simulink model "Final_Simulation_unfiltered_speed"  (R2024b)
settings: Solver=VariableStepAuto  StartTime=0.0  StopTime=30  MaxStep=1e-4  RelTol=1e-4
libraries: spsDiodeLib x7, spsVoltageMeasurementLib x5, spsCurrentMeasurementLib x4, spsControlledVoltageSourceLib x3, spsDCMachineLib x1, spsDCVoltageSourceLib x1, spsGroundLib x1, spsMosfetLib x1, slpidlib x1, spsPWMGeneratorDCDCLib x1, spsRMSLib x1, spsSeriesRLCBranchLib x1
settings Model: Creator=sefer  LastModifiedBy=PC
settings DebuggingCC: IgnoredZcDiagnostic=none

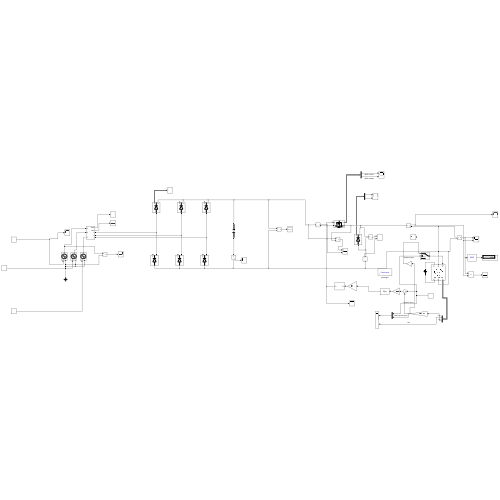
[thumbnail: Simulink's stored preview of the top-level diagram]
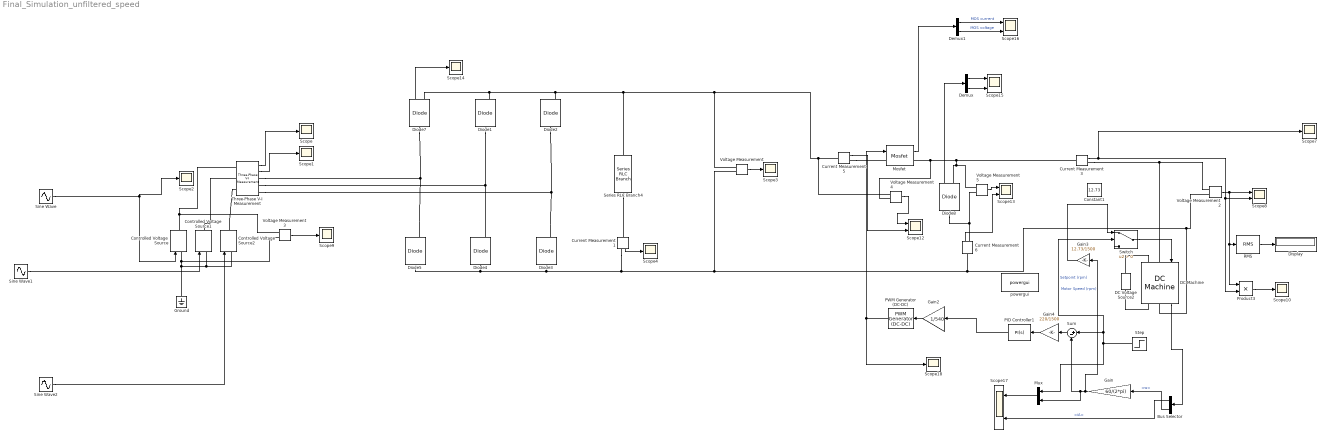
== system Final_Simulation_unfiltered_speed ==
  Bus Selector : BusSelector  OutputSignals=iA,w
  Constant1 : Constant  Value=12.73
  Controlled Voltage Source : spsControlledVoltageSourceLib/Controlled Voltage Source  Initialize=on  Source_Type=AC  Amplitude=0  Phase=0  Frequency=50  Measurements=None
  Controlled Voltage Source1 : spsControlledVoltageSourceLib/Controlled Voltage Source  Initialize=on  Source_Type=AC  Amplitude=0  Phase=0  Frequency=50  Measurements=None
  Controlled Voltage Source2 : spsControlledVoltageSourceLib/Controlled Voltage Source  Initialize=on  Source_Type=AC  Amplitude=0  Phase=0  Frequency=50  Measurements=None
  Current Measurement{1,3,5..6} (4 alike) : spsCurrentMeasurementLib/Current Measurement  PhasorSimulation=off  OutputType=Complex  PSBequivalent=0
  DC Machine : spsDCMachineLib/DC Machine  PresetModel=No  MechanicalLoad=Torque TL  FieldType=Wound  ShowDetailedParameters=on  MeasurementBus=on  RLa="[ 0.8  12.5e-3]"  RLf="[210  23]"  Laf=1.3  MachineConstant=Torque constant (N.m/A)  Ke=1.8  Kt=1.8  J=0.2  Bm=0.005  Tf=0  w0=0  Ifinit=1.04761904761905  TsPowergui=0  TsBlock=-1
  DC Voltage Source2 : spsDCVoltageSourceLib/DC Voltage Source  Amplitude=220  Measurements=None
  Demux : Demux  Outputs=2
  Demux1 : Demux  Outputs=2
  Diode{1..5,7} (6 alike) : spsDiodeLib/Diode  Ron=0.001  Lon=0  Vf=0  IC=0  UseSnubber=0  Rs=inf  Cs=0  Measurements=on
  Diode8 : spsDiodeLib/Diode  Ron=0  Lon=0  Vf=0  IC=0  UseSnubber=0  Rs=inf  Cs=0  Measurements=on
  Display : Display
  Gain : Gain  Gain=60/(2*pi)
  Gain2 : Gain  Gain=1/540
  Gain3 : Gain  Gain=12.73/1500
  Gain4 : Gain  Gain=220/1500
  Ground : spsGroundLib/Ground  LConnTagsString=a
  Mosfet : spsMosfetLib/Mosfet  Ron=0.1  Lon=0  Rd=0.01  Vfd=0  IC=0  Rs=1e5  Cs=inf  Measurements=on
  Mux : Mux  Inputs=2
  PID Controller1 : slpidlib/PID Controller  Controller=PI  Form=Parallel  TimeDomain=Continuous-time  UseExternalTs=off  SampleTime=-1  IntegratorMethod=Forward Euler  FilterMethod=Forward Euler  ControllerParametersSource=internal  P=0.01  I=0.28994889807594  UseKiTs=off  D=-0.000982857561820016  UseExternalDerivativeSource=off  N=2.14059506099866  UseFilter=on  TunerSelectOption=Transfer Function Based (PID Tuner App)  InitialConditionSource=internal  InitialConditionForIntegrator=0  InitialConditionForFilter=0  DifferentiatorICPrevScaledInput=0  ExternalReset=none  TrackingMode=off  Kt=1  LimitOutput=off  SatLimitsSource=internal  UpperSaturationLimit=100  LowerSaturationLimit=-100  LinearizeAsGain=on  AntiWindupMode=none  Kb=1  LimitIntegrator=on  UpperIntegratorSaturationLimit=1500  LowerIntegratorSaturationLimit=-1500  POutMin=[]  POutMax=[]  IOutMin=[]  IOutMax=[]  DOutMin=[]  DOutMax=[]  NOutMin=[]  NOutMax=[]  SumOutMin=[]  SumOutMax=[]  SaturationOutMin=[]  SaturationOutMax=[]  PParamMin=[]  PParamMax=[]  IParamMin=[]  IParamMax=[]  DParamMin=[]  DParamMax=[]  NParamMin=[]  NParamMax=[]  KbParamMin=[]  KbParamMax=[]  KtParamMin=[]  KtParamMax=[]  KbOutMin=[]  KbOutMax=[]  KtOutMin=[]  KtOutMax=[]  IntegratorOutMin=[]  IntegratorOutMax=[]  FilterOutMin=[]  FilterOutMax=[]  SumI1OutMin=[]  SumI1OutMax=[]  SumI2OutMin=[]  SumI2OutMax=[]  SumI3OutMin=[]  SumI3OutMax=[]  SumI4OutMin=[]  SumI4OutMax=[]  SumDOutMin=[]  SumDOutMax=[]  DifferentiatorOutMin=[]  DifferentiatorOutMax=[]  FilterDiffOutCoefMin=[]  FilterDiffOutCoefMax=[]  ReciprocalOutMin=[]  ReciprocalOutMax=[]  SumDenOutMin=[]  SumDenOutMax=[]  SumNumOutMin=[]  SumNumOutMax=[]  DivideOutMin=[]  DivideOutMax=[]  UdiffTsProdOutMin=[]  UdiffTsProdOutMax=[]  NTsProdOutMin=[]  NTsProdOutMax=[]  UintegralTsProdOutMin=[]  UintegralTsProdOutMax=[]  UngainTsProdOutMin=[]  UngainTsProdOutMax=[]  ClampingZeroOutDataTypeStr=Inherit: Inherit via back propagation  ClampingZeroOutMin=[]  ClampingZeroOutMax=[]  FilterDenConstantOutDataTypeStr=Inherit: Inherit via back propagation  FilterDenConstantOutMin=[]  FilterDenConstantOutMax=[]  PCopyOutDataTypeStr=Inherit: Inherit via back propagation  PCopyOutMin=[]  PCopyOutMax=[]  NCopyOutDataTypeStr=Inherit: Inherit via back propagation  NCopyOutMin=[]  NCopyOutMax=[]  IntegratorContinuousStateAttributes=''  IntegratorStateMustResolveToSignalObject=off  IntegratorRTWStateStorageClass=Auto  FilterContinuousStateAttributes=''  FilterStateMustResolveToSignalObject=off  FilterRTWStateStorageClass=Auto  ParallelPVariant=InternalParameters  IdealPVariant=Disabled  IVariant=InternalParameters  DVariant=Disabled  IntegratorVariant=Continuous  SatVariant=Disabled  AWVariant=Passthrough  PCopyVariant=Disabled  TRVariant=Disabled  FdbkBlocksVariant=Forward  IdealPFdbkVariant=Disabled  SatFdbkVariant=Disabled  DerivativeFilterVariant=Disabled  NVariant=Disabled  NCopyVariant=Disabled_SignalSpec  FilterICVariant=Disabled  IntegratorICVariant=InternalICs  ExternalResetVariant=Disabled  TRSumVariant=Passthrough  SumFdbkVariant=Disabled  SumVariant=Sum_PI  TsampFilterVariant=InternalTs  TsampNgainVariant=Passthrough  TsampIntegralVariant=Disabled_SignalSpec  ExternalSaturationOutDataTypeStr=Inherit: Same as second input  DerivativeSourceVariant=Disabled  PreIntVariant=InternalPreInt
  PWM Generator (DC-DC) : spsPWMGeneratorDCDCLib/PWM Generator (DC-DC)  Fsw=5000  Ts=0
  Product3 : Product
  RMS : spsRMSLib/RMS  TrueRMS=on  Freq=60  RMSInit=120  Ts=0
  Scope{,1..4,7,9..10,14,18} (10 alike) : Scope
  Scope{8,12..13,15..17} (6 alike) : Scope  NumInputPorts=2
  Series RLC Branch4 : spsSeriesRLCBranchLib/Series RLC Branch  LConnTagsString=__new0  RConnTagsString=__new0  BranchType=C  Resistance=0.001  Inductance=1e-3  SetiL0=off  InitialCurrent=0  Capacitance=2000e-6  Setx0=off  InitialVoltage=0  Measurements=None
  Sine Wave : Sin  Amplitude=230*sqrt(2)  Frequency=100*pi  SampleTime=0
  Sine Wave1 : Sin  Amplitude=230*sqrt(2)  Frequency=100*pi  Phase=2*pi/3  SampleTime=0
  Sine Wave2 : Sin  Amplitude=230*sqrt(2)  Frequency=100*pi  Phase=4*pi/3  SampleTime=0
  Step : Step  After=1500  SampleTime=0
  Sum : Sum  Inputs=|+-
  Switch : Switch  Criteria=u2 > Threshold  SaturateOnIntegerOverflow=off  InputSameDT=off
  Three-Phase V-I Measurement : spsThreePhaseVIMeasurementLib/Three-Phase V-I Measurement  VoltageMeasurement=phase-to-ground  SetLabelV=off  LabelV=Vabc  Vpu=off  VpuLL=off  CurrentMeasurement=yes  SetLabelI=off  LabelI=Iabc  Ipu=off  Pbase=100e6  Vbase=500e3  OutputType=Complex  PhasorSimulation=off  PSBequivalent=0
  Voltage Measurement{,2..5} (5 alike) : spsVoltageMeasurementLib/Voltage Measurement  PhasorSimulation=off  OutputType=Complex  PSBequivalent=0
  powergui : sps_lib/powergui  Priority=1  SimulationMode=Continuous  SampleTime=1e-6  frequency=60  Iterations=50  frequencyindice=0  Pbase=100e6  ErrMax=1e-4  UnitsV=kV  UnitsW=MW  buscounter=0  FunctionMessages=off  echomessages=off  EnableUseOfTLC=off  CurrentSourceSwitches=off  DisableSnubberDevices=off  DisableRonSwitches=off  DisableVfSwitches=off  DisplayEquations=off  AutomaticDiscreteSolvers=off  SolverType=Tustin/Backward Euler (TBE)  Interpol=off  ExternalGateDelay=off  methode=off  Ts=100  x0status=blocks  SPID=on  SwTol=0  HookPort=off  NonlinearTolerance=1e-4  nMaxIteration=100  ContinueOnMaxIteration=off  RestoreLinks=warning  ResistiveCurrentMeasurement=off  Frange=[0:2:500]  Ylog=off  Xlog=on  ShowGrid=off  save=off  variable=ZData  structure=0  ZoomFFT=off  StartTime=0.0  cycles=1  DisplayStyle=1  fundamental=60  FreqAxis=off  MaxFrequency=1000  frequencyindicesteady=1  RmsSteady=1  display=off
  wires:
  Three-Phase V-I Measurement/1 -> Scope/1
  Three-Phase V-I Measurement/2 -> Scope1/1
  Voltage Measurement/1 -> Scope3/1
  Current Measurement1/1 -> Scope4/1
  Voltage Measurement2/1 -> Product3/1, RMS/1, Scope8/1
  Voltage Measurement3/1 -> Scope9/1
  Sine Wave/1 -> Scope2/1, Controlled Voltage Source/1
  RMS/1 -> Display/1
  Product3/1 -> Scope10/1
  PWM Generator (DC-DC)/1 -> Scope18/1, Mosfet/1
  Sine Wave1/1 -> Controlled Voltage Source1/1
  Sine Wave2/1 -> Controlled Voltage Source2/1
  Voltage Measurement4/1 -> Scope12/1
  Voltage Measurement5/1 -> Scope13/1
  Current Measurement5/1 -> Scope12/2
  Current Measurement6/1 -> Scope13/2
  Diode7/1 -> Scope14/1
  Diode8/1 -> Demux/1
  Demux/1 -> Scope15/1
  Demux/2 -> Scope15/2
  Demux1/1 -> Scope16/1  "MOS current"
  Demux1/2 -> Scope16/2  "MOS voltage"
  Mosfet/1 -> Demux1/1
  DC Machine/1 -> Bus Selector/1
  Gain/1 -> Gain3/1, Sum/2, Mux/2  "Motor Speed (rpm)"
  Step/1 -> Switch/2, Sum/1, Mux/1  "Setpoint (rpm)"
  Mux/1 -> Scope17/1
  Current Measurement3/1 -> Scope8/2, Product3/2, Scope7/1
  Bus Selector/1 -> Scope17/2  "<iA>"
  Gain2/1 -> PWM Generator (DC-DC)/1
  Bus Selector/2 -> Gain/1  "<w>"
  Switch/1 -> DC Machine/1
  Sum/1 -> Gain4/1
  Gain4/1 -> PID Controller1/1
  PID Controller1/1 -> Gain2/1
  Gain3/1 -> Switch/1
  connections:
  Diode5/RConn1 -- Three-Phase V-I Measurement/RConn1 -- Diode7/LConn1
  Diode4/RConn1 -- Three-Phase V-I Measurement/RConn2 -- Diode1/LConn1
  Series RLC Branch4/RConn1 -- Current Measurement1/LConn1
  Diode1/RConn1 -- Diode7/RConn1 -- Diode2/RConn1 -- Voltage Measurement4/LConn1 -- Current Measurement5/LConn1 -- Voltage Measurement/LConn1 -- Series RLC Branch4/LConn1
  Diode3/RConn1 -- Three-Phase V-I Measurement/RConn3 -- Diode2/LConn1
  Diode8/RConn1 -- Voltage Measurement5/LConn1 -- Current Measurement3/LConn1 -- Voltage Measurement4/LConn2 -- Mosfet/RConn1
  Current Measurement3/RConn1 -- DC Machine/LConn1 -- Voltage Measurement2/LConn1
  Voltage Measurement2/LConn2 -- DC Machine/RConn1 -- Current Measurement6/LConn1 -- Diode3/LConn1 -- Diode5/LConn1 -- Diode4/LConn1 -- Current Measurement1/RConn1 -- Voltage Measurement/LConn2
  Ground/LConn1 -- Voltage Measurement3/LConn2 -- Controlled Voltage Source/LConn1 -- Controlled Voltage Source2/LConn1 -- Controlled Voltage Source1/LConn1
  Controlled Voltage Source/RConn1 -- Voltage Measurement3/LConn1 -- Three-Phase V-I Measurement/LConn1
  Controlled Voltage Source1/RConn1 -- Three-Phase V-I Measurement/LConn2
  Controlled Voltage Source2/RConn1 -- Three-Phase V-I Measurement/LConn3
  DC Voltage Source2/RConn1 -- DC Machine/LConn2
  DC Voltage Source2/LConn1 -- DC Machine/RConn2
  Current Measurement5/RConn1 -- Mosfet/LConn1
  Voltage Measurement5/LConn2 -- Diode8/LConn1 -- Current Measurement6/RConn1
